simulink library "MBDS_Applications"  (R2018b)
settings: Solver=ode45  StartTime=0.0  StopTime=10.0  RelTol=1e-3
undefined symbols (not defined in the file or in its folder): Ts
libraries: KIBES_Signal x297, simulink x7
(part 5 of 6)

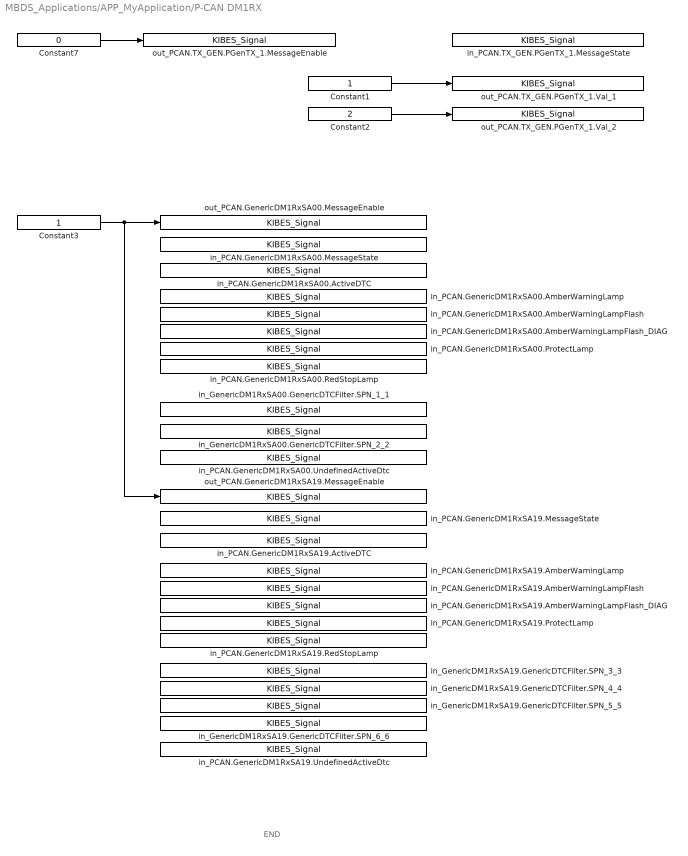
== system MBDS_Applications/APP_MyApplication/P-CAN DM1RX ==
  note: END
  Constant1 : Constant  InitFcn=|  OutDataTypeStr=uint8
      | if(exist('MBDS_BlockCallback', 'file'))
      |    MBDS_BlockCallback('Update', gcb);  
      | end
  Constant2 : Constant  InitFcn=|  Value=2  OutDataTypeStr=uint8
      | if(exist('MBDS_BlockCallback', 'file'))
      |    MBDS_BlockCallback('Update', gcb);  
      | end
  Constant3 : Constant  InitFcn=|  OutDataTypeStr=boolean
      | if(exist('MBDS_BlockCallback', 'file'))
      |    MBDS_BlockCallback('Update', gcb);  
      | end
  Constant7 : Constant  InitFcn=|  Value=0  OutDataTypeStr=boolean
      | if(exist('MBDS_BlockCallback', 'file'))
      |    MBDS_BlockCallback('Update', gcb);  
      | end
  in_GenericDM1RxSA00.GenericDTCFilter.SPN_1_1 : KIBES_Signal/KIBES_Signal  MBDS_LibraryBlock=on  DatabaseKey=293  SignalName=GenericDM1RxSA00.GenericDTCFilter.SPN_1_1  SymbolName=GenericDM1RxSA00_GenericDTCFilter_SPN_1_1_000293  DataType=boolean  Init=0  Slope=1  Bias=0  DataSize=1  fpDataType=boolean  BlockIOType=Inport  DeviceType=0
  in_GenericDM1RxSA00.GenericDTCFilter.SPN_2_2 : KIBES_Signal/KIBES_Signal  MBDS_LibraryBlock=on  DatabaseKey=294  SignalName=GenericDM1RxSA00.GenericDTCFilter.SPN_2_2  SymbolName=GenericDM1RxSA00_GenericDTCFilter_SPN_2_2_000294  DataType=boolean  Init=0  Slope=1  Bias=0  DataSize=1  fpDataType=boolean  BlockIOType=Inport  DeviceType=0
  in_GenericDM1RxSA19.GenericDTCFilter.SPN_3_3 : KIBES_Signal/KIBES_Signal  MBDS_LibraryBlock=on  DatabaseKey=290  SignalName=GenericDM1RxSA19.GenericDTCFilter.SPN_3_3  SymbolName=GenericDM1RxSA19_GenericDTCFilter_SPN_3_3_000290  DataType=boolean  Init=0  Slope=1  Bias=0  DataSize=1  fpDataType=boolean  BlockIOType=Inport  DeviceType=0
  in_GenericDM1RxSA19.GenericDTCFilter.SPN_4_4 : KIBES_Signal/KIBES_Signal  MBDS_LibraryBlock=on  DatabaseKey=291  SignalName=GenericDM1RxSA19.GenericDTCFilter.SPN_4_4  SymbolName=GenericDM1RxSA19_GenericDTCFilter_SPN_4_4_000291  DataType=boolean  Init=0  Slope=1  Bias=0  DataSize=1  fpDataType=boolean  BlockIOType=Inport  DeviceType=0
  in_GenericDM1RxSA19.GenericDTCFilter.SPN_5_5 : KIBES_Signal/KIBES_Signal  MBDS_LibraryBlock=on  DatabaseKey=296  SignalName=GenericDM1RxSA19.GenericDTCFilter.SPN_5_5  SymbolName=GenericDM1RxSA19_GenericDTCFilter_SPN_5_5_000296  DataType=boolean  Init=0  Slope=1  Bias=0  DataSize=1  fpDataType=boolean  BlockIOType=Inport  DeviceType=0
  in_GenericDM1RxSA19.GenericDTCFilter.SPN_6_6 : KIBES_Signal/KIBES_Signal  MBDS_LibraryBlock=on  DatabaseKey=303  SignalName=GenericDM1RxSA19.GenericDTCFilter.SPN_6_6  SymbolName=GenericDM1RxSA19_GenericDTCFilter_SPN_6_6_000303  DataType=boolean  Init=0  Slope=1  Bias=0  DataSize=1  fpDataType=boolean  BlockIOType=Inport  DeviceType=0
  in_PCAN.GenericDM1RxSA00.ActiveDTC : KIBES_Signal/KIBES_Signal  MBDS_LibraryBlock=on  DatabaseKey=274  SignalName=PCAN.GenericDM1RxSA00.ActiveDTC  SymbolName=PCAN_GenericDM1RxSA00_ActiveDTC_000274  DataType=boolean  Init=0  Slope=1  Bias=0  DataSize=1  fpDataType=boolean  BlockIOType=Inport  DeviceType=0
  in_PCAN.GenericDM1RxSA00.AmberWarningLamp : KIBES_Signal/KIBES_Signal  MBDS_LibraryBlock=on  DatabaseKey=275  SignalName=PCAN.GenericDM1RxSA00.AmberWarningLamp  SymbolName=PCAN_GenericDM1RxSA00_AmberWarningLamp_000275  DataType=boolean  Init=0  Slope=1  Bias=0  DataSize=1  fpDataType=boolean  BlockIOType=Inport  DeviceType=0
  in_PCAN.GenericDM1RxSA00.AmberWarningLampFlash : KIBES_Signal/KIBES_Signal  MBDS_LibraryBlock=on  DatabaseKey=276  SignalName=PCAN.GenericDM1RxSA00.AmberWarningLampFlash  SymbolName=PCAN_GenericDM1RxSA00_AmberWarningLampFlash_000276  DataType=uint8  Init=0  Slope=1  Bias=0  DataSize=1  fpDataType=uint8  BlockIOType=Inport  DeviceType=0
  in_PCAN.GenericDM1RxSA00.AmberWarningLampFlash_DIAG : KIBES_Signal/KIBES_Signal  MBDS_LibraryBlock=on  DatabaseKey=277  SignalName=PCAN.GenericDM1RxSA00.AmberWarningLampFlash_DIAG  SymbolName=PCAN_GenericDM1RxSA00_AmberWarningLampFlash_DIAG_000277  DataType=uint16  Init=1  Slope=1  Bias=0  DataSize=1  fpDataType=uint16  BlockIOType=Inport  DeviceType=0
  in_PCAN.GenericDM1RxSA00.MessageState : KIBES_Signal/KIBES_Signal  MBDS_LibraryBlock=on  DatabaseKey=279  SignalName=PCAN.GenericDM1RxSA00.MessageState  SymbolName=PCAN_GenericDM1RxSA00_MessageState_000279  DataType=uint16  Init=0  Slope=1  Bias=0  DataSize=1  fpDataType=uint16  BlockIOType=Inport  DeviceType=0
  in_PCAN.GenericDM1RxSA00.ProtectLamp : KIBES_Signal/KIBES_Signal  MBDS_LibraryBlock=on  DatabaseKey=280  SignalName=PCAN.GenericDM1RxSA00.ProtectLamp  SymbolName=PCAN_GenericDM1RxSA00_ProtectLamp_000280  DataType=boolean  Init=0  Slope=1  Bias=0  DataSize=1  fpDataType=boolean  BlockIOType=Inport  DeviceType=0
  in_PCAN.GenericDM1RxSA00.RedStopLamp : KIBES_Signal/KIBES_Signal  MBDS_LibraryBlock=on  DatabaseKey=281  SignalName=PCAN.GenericDM1RxSA00.RedStopLamp  SymbolName=PCAN_GenericDM1RxSA00_RedStopLamp_000281  DataType=boolean  Init=0  Slope=1  Bias=0  DataSize=1  fpDataType=boolean  BlockIOType=Inport  DeviceType=0
  in_PCAN.GenericDM1RxSA00.UndefinedActiveDtc : KIBES_Signal/KIBES_Signal  MBDS_LibraryBlock=on  DatabaseKey=403  SignalName=PCAN.GenericDM1RxSA00.UndefinedActiveDtc  SymbolName=PCAN_GenericDM1RxSA00_UndefinedActiveDtc_000403  DataType=boolean  Init=0  Slope=1  Bias=0  DataSize=1  fpDataType=boolean  BlockIOType=Inport  DeviceType=0
  in_PCAN.GenericDM1RxSA19.ActiveDTC : KIBES_Signal/KIBES_Signal  MBDS_LibraryBlock=on  DatabaseKey=282  SignalName=PCAN.GenericDM1RxSA19.ActiveDTC  SymbolName=PCAN_GenericDM1RxSA19_ActiveDTC_000282  DataType=boolean  Init=0  Slope=1  Bias=0  DataSize=1  fpDataType=boolean  BlockIOType=Inport  DeviceType=0
  in_PCAN.GenericDM1RxSA19.AmberWarningLamp : KIBES_Signal/KIBES_Signal  MBDS_LibraryBlock=on  DatabaseKey=283  SignalName=PCAN.GenericDM1RxSA19.AmberWarningLamp  SymbolName=PCAN_GenericDM1RxSA19_AmberWarningLamp_000283  DataType=boolean  Init=0  Slope=1  Bias=0  DataSize=1  fpDataType=boolean  BlockIOType=Inport  DeviceType=0
  in_PCAN.GenericDM1RxSA19.AmberWarningLampFlash : KIBES_Signal/KIBES_Signal  MBDS_LibraryBlock=on  DatabaseKey=284  SignalName=PCAN.GenericDM1RxSA19.AmberWarningLampFlash  SymbolName=PCAN_GenericDM1RxSA19_AmberWarningLampFlash_000284  DataType=uint8  Init=0  Slope=1  Bias=0  DataSize=1  fpDataType=uint8  BlockIOType=Inport  DeviceType=0
  in_PCAN.GenericDM1RxSA19.AmberWarningLampFlash_DIAG : KIBES_Signal/KIBES_Signal  MBDS_LibraryBlock=on  DatabaseKey=285  SignalName=PCAN.GenericDM1RxSA19.AmberWarningLampFlash_DIAG  SymbolName=PCAN_GenericDM1RxSA19_AmberWarningLampFlash_DIAG_000285  DataType=uint16  Init=1  Slope=1  Bias=0  DataSize=1  fpDataType=uint16  BlockIOType=Inport  DeviceType=0
  in_PCAN.GenericDM1RxSA19.MessageState : KIBES_Signal/KIBES_Signal  MBDS_LibraryBlock=on  DatabaseKey=287  SignalName=PCAN.GenericDM1RxSA19.MessageState  SymbolName=PCAN_GenericDM1RxSA19_MessageState_000287  DataType=uint16  Init=0  Slope=1  Bias=0  DataSize=1  fpDataType=uint16  BlockIOType=Inport  DeviceType=0
  in_PCAN.GenericDM1RxSA19.ProtectLamp : KIBES_Signal/KIBES_Signal  MBDS_LibraryBlock=on  DatabaseKey=288  SignalName=PCAN.GenericDM1RxSA19.ProtectLamp  SymbolName=PCAN_GenericDM1RxSA19_ProtectLamp_000288  DataType=boolean  Init=0  Slope=1  Bias=0  DataSize=1  fpDataType=boolean  BlockIOType=Inport  DeviceType=0
  in_PCAN.GenericDM1RxSA19.RedStopLamp : KIBES_Signal/KIBES_Signal  MBDS_LibraryBlock=on  DatabaseKey=289  SignalName=PCAN.GenericDM1RxSA19.RedStopLamp  SymbolName=PCAN_GenericDM1RxSA19_RedStopLamp_000289  DataType=boolean  Init=0  Slope=1  Bias=0  DataSize=1  fpDataType=boolean  BlockIOType=Inport  DeviceType=0
  in_PCAN.GenericDM1RxSA19.UndefinedActiveDtc : KIBES_Signal/KIBES_Signal  MBDS_LibraryBlock=on  DatabaseKey=404  SignalName=PCAN.GenericDM1RxSA19.UndefinedActiveDtc  SymbolName=PCAN_GenericDM1RxSA19_UndefinedActiveDtc_000404  DataType=boolean  Init=0  Slope=1  Bias=0  DataSize=1  fpDataType=boolean  BlockIOType=Inport  DeviceType=0
  in_PCAN.TX_GEN.PGenTX_1.MessageState : KIBES_Signal/KIBES_Signal  MBDS_LibraryBlock=on  DatabaseKey=260  SignalName=PCAN.TX_GEN.PGenTX_1.MessageState  SymbolName=PCAN_TX_GEN_PGenTX_1_MessageState_000260  DataType=uint16  Init=0  Slope=1  Bias=0  DataSize=1  fpDataType=uint16  BlockIOType=Inport  DeviceType=0
  out_PCAN.GenericDM1RxSA00.MessageEnable : KIBES_Signal/KIBES_Signal  MBDS_LibraryBlock=on  DatabaseKey=278  SignalName=PCAN.GenericDM1RxSA00.MessageEnable  SymbolName=PCAN_GenericDM1RxSA00_MessageEnable_000278  DataType=boolean  Init=0  Slope=1  Bias=0  DataSize=1  fpDataType=boolean  BlockIOType=Outport  DeviceType=0
  out_PCAN.GenericDM1RxSA19.MessageEnable : KIBES_Signal/KIBES_Signal  MBDS_LibraryBlock=on  DatabaseKey=286  SignalName=PCAN.GenericDM1RxSA19.MessageEnable  SymbolName=PCAN_GenericDM1RxSA19_MessageEnable_000286  DataType=boolean  Init=0  Slope=1  Bias=0  DataSize=1  fpDataType=boolean  BlockIOType=Outport  DeviceType=0
  out_PCAN.TX_GEN.PGenTX_1.MessageEnable : KIBES_Signal/KIBES_Signal  MBDS_LibraryBlock=on  DatabaseKey=259  SignalName=PCAN.TX_GEN.PGenTX_1.MessageEnable  SymbolName=PCAN_TX_GEN_PGenTX_1_MessageEnable_000259  DataType=boolean  Init=0  Slope=1  Bias=0  DataSize=1  fpDataType=boolean  BlockIOType=Outport  DeviceType=0
  out_PCAN.TX_GEN.PGenTX_1.Val_1 : KIBES_Signal/KIBES_Signal  MBDS_LibraryBlock=on  DatabaseKey=261  SignalName=PCAN.TX_GEN.PGenTX_1.Val_1  SymbolName=PCAN_TX_GEN_PGenTX_1_Val_1_000261  DataType=uint8  Init=0  Slope=1  Bias=0  DataSize=1  fpDataType=uint8  BlockIOType=Outport  DeviceType=0
  out_PCAN.TX_GEN.PGenTX_1.Val_2 : KIBES_Signal/KIBES_Signal  MBDS_LibraryBlock=on  DatabaseKey=262  SignalName=PCAN.TX_GEN.PGenTX_1.Val_2  SymbolName=PCAN_TX_GEN_PGenTX_1_Val_2_000262  DataType=uint8  Init=0  Slope=1  Bias=0  DataSize=1  fpDataType=uint8  BlockIOType=Outport  DeviceType=0
  wires:
  Constant3/1 -> out_PCAN.GenericDM1RxSA00.MessageEnable/1, out_PCAN.GenericDM1RxSA19.MessageEnable/1
  Constant2/1 -> out_PCAN.TX_GEN.PGenTX_1.Val_2/1
  Constant1/1 -> out_PCAN.TX_GEN.PGenTX_1.Val_1/1
  Constant7/1 -> out_PCAN.TX_GEN.PGenTX_1.MessageEnable/1

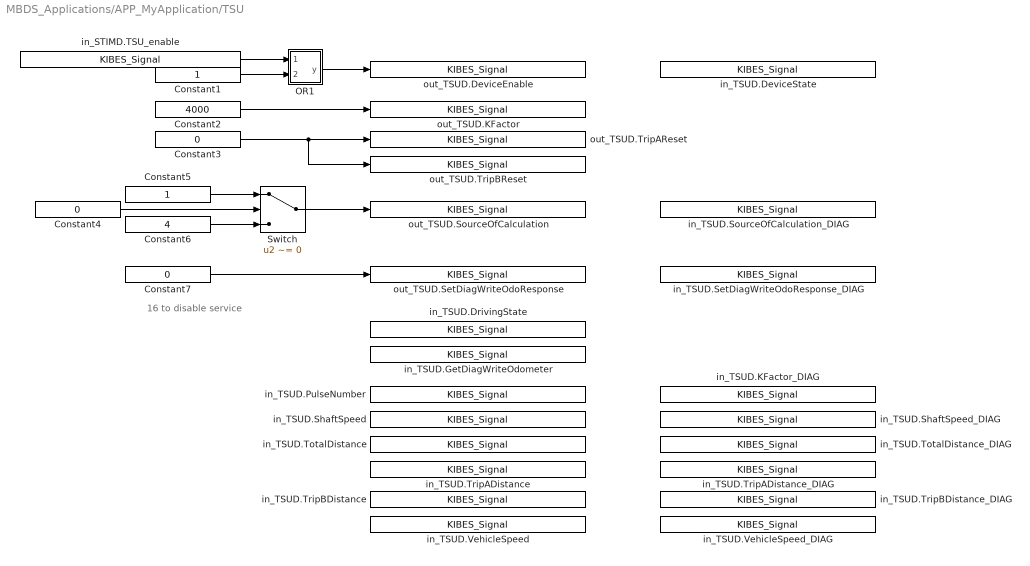
== system MBDS_Applications/APP_MyApplication/TSU ==
  note: 16 to disable service
  Constant1 : Constant  InitFcn=|  OutDataTypeStr=boolean
      | if(exist('MBDS_BlockCallback', 'file'))
      |    MBDS_BlockCallback('Update', gcb);  
      | end
  Constant2 : Constant  InitFcn=|  Value=4000  OutDataTypeStr=uint32
      | if(exist('MBDS_BlockCallback', 'file'))
      |    MBDS_BlockCallback('Update', gcb);  
      | end
  Constant3 : Constant  InitFcn=|  Value=0  OutDataTypeStr=boolean
      | if(exist('MBDS_BlockCallback', 'file'))
      |    MBDS_BlockCallback('Update', gcb);  
      | end
  Constant4 : Constant  InitFcn=|  Value=0  OutDataTypeStr=boolean
      | if(exist('MBDS_BlockCallback', 'file'))
      |    MBDS_BlockCallback('Update', gcb);  
      | end
  Constant5 : Constant  InitFcn=|  OutDataTypeStr=uint8
      | if(exist('MBDS_BlockCallback', 'file'))
      |    MBDS_BlockCallback('Update', gcb);  
      | end
  Constant6 : Constant  InitFcn=|  Value=4  OutDataTypeStr=uint8
      | if(exist('MBDS_BlockCallback', 'file'))
      |    MBDS_BlockCallback('Update', gcb);  
      | end
  Constant7 : Constant  InitFcn=|  Value=0  OutDataTypeStr=uint8
      | if(exist('MBDS_BlockCallback', 'file'))
      |    MBDS_BlockCallback('Update', gcb);  
      | end
  OR1 : Subsystem  InitFcn=|  mask(OR){MBDS_LibraryBlock=on, BitwiseMode=off, Inputs=2, UseBitMask=off, BitMask='A1', OutDataTypeStr=Inherit: Inherit via back propagation, MBDS_BlockVersion=07.21.05}
      | if(exist('MBDS_BlockCallback', 'file'))
      |    MBDS_BlockCallback('Update', gcb);
      | end
      mask prompts: MBDS_LibraryBlock "MBDS library block"; BitwiseMode "Use 'bitwise' mode"; Inputs "Number of input ports:"; UseBitMask "Use bit mask"; BitMask "Bit mask:"; OutDataTypeStr "Output data type:"; MBDS_BlockVersion "Version:"
      mask help: Logical or bitwise OR operator. For multiple inputs, operators are applied across the inputs. For a single input, operators are applied across the input vector. In bitwise mode a bit mask can be applied onto single input signals.
      mask init: same as MBDS_Applications/APP_MyApplication/NOT
      mask Help: eval(['open([workdir(''library_dir:''),''\Blockset\help\'',get_param(gcb,''MaskType''),''.html''])'])
      mask Callback BitwiseMode:
      | if(exist('MBDS_BlockCallback', 'file'))
      |    MBDS_BlockCallback('BitwiseMode', gcb);
      | end
      mask Callback Inputs:
      | if(exist('MBDS_BlockCallback', 'file'))
      |    MBDS_BlockCallback('Inputs', gcb);
      | end
      mask Callback UseBitMask:
      | if(exist('MBDS_BlockCallback', 'file'))
      |    MBDS_BlockCallback('UseBitMask', gcb);
      | end
      mask Callback BitMask:
      | if(exist('MBDS_BlockCallback', 'file'))
      |    MBDS_BlockCallback('BitMask', gcb);
      | end
      mask TypeOptions OutDataTypeStr: Inherit: Inherit via back propagation | int8 | uint8 | int16 | uint16 | int32 | uint32 | boolean
      mask Callback OutDataTypeStr:
      | % Adopt Value
      | if(exist('MBDS_BlockCallback', 'file'))
      |    MBDS_BlockCallback('OutDataTypeStr', gcb);
      | end
      mask DialogControl ParameterTabVar0 Prompt: Main
      mask DialogControl ParameterTabVar01 Prompt: Signal Attributes
      mask DialogControl ParameterTabVar012 Prompt: Version
      mask Display:
      | % Show icon or block text
      | if(UseBitMask)
      |    if(isnumeric(BitMask))
      |       BitMaskString = ['0x',dec2hex(floor(BitMask))];
      |    elseif(ischar(BitMask))
      |       BitMaskString = ['0x',upper(BitMask)];
      |    else
      |       BitMaskString = '???';
      |    end
      |    disp(sprintf(['OR\n', BitMaskString]))
      | else
      |    disp('OR')
      | end
  Switch : Switch  InitFcn=|  Criteria=u2 ~= 0  OutDataTypeStr=Inherit: Inherit via back propagation  mask(Switch){MBDS_LibraryBlock=on, OutDataTypeStr_=Inherit: Inherit via back propagation, SaturateOnIntegerOverflow_=off, InputSameDT_=off, MBDS_BlockVersion=07.21.05}
      | if(exist('MBDS_BlockCallback', 'file'))
      |    MBDS_BlockCallback('Update', gcb);  
      | end
      mask prompts: MBDS_LibraryBlock "MBDS library block"; OutDataTypeStr_ "Output data type:"; SaturateOnIntegerOverflow_ "Saturate on integer overflow"; InputSameDT_ "Require all inputs to have the same data type"; MBDS_BlockVersion "Block version:"
      mask help: Pass through input 1 when input 2 is not equal to zero; otherwise pass through input 3. The inputs are numbered top to bottom (or left to right). The first and third input ports are data ports, and the second input port is the control port.
      mask init: same as MBDS_Applications/APP_MyApplication/NOT
      mask Help: eval(['open([workdir(''library_dir:''),''\Blockset\help\'',get_param(gcb,''MaskType''),''.html''])'])
      mask TypeOptions OutDataTypeStr_: Inherit: Inherit via back propagation | single | int8 | uint8 | int16 | uint16 | int32 | uint32
      mask DialogControl ParameterTabVar0 Prompt: Signal Attributes
      mask DialogControl ParameterTabVar01 Prompt: Version
  in_STIMD.TSU_enable : KIBES_Signal/KIBES_Signal  MBDS_LibraryBlock=on  DatabaseKey=391  SignalName=STIMD.TSU_enable  SymbolName=STIMD_TSU_enable_000391  DataType=boolean  Init=0  Slope=1  Bias=0  DataSize=1  fpDataType=boolean  BlockIOType=Inport  DeviceType=2
  in_TSUD.DeviceState : KIBES_Signal/KIBES_Signal  MBDS_LibraryBlock=on  DatabaseKey=379  SignalName=TSUD.DeviceState  SymbolName=TSUD_DeviceState_000379  DataType=uint16  Init=0  Slope=1  Bias=0  DataSize=1  fpDataType=uint16  BlockIOType=Inport  DeviceType=0
  in_TSUD.DrivingState : KIBES_Signal/KIBES_Signal  MBDS_LibraryBlock=on  DatabaseKey=376  SignalName=TSUD.DrivingState  SymbolName=TSUD_DrivingState_000376  DataType=boolean  Init=0  Slope=1  Bias=0  DataSize=1  fpDataType=boolean  BlockIOType=Inport  DeviceType=0
  in_TSUD.GetDiagWriteOdometer : KIBES_Signal/KIBES_Signal  MBDS_LibraryBlock=on  DatabaseKey=383  SignalName=TSUD.GetDiagWriteOdometer  SymbolName=TSUD_GetDiagWriteOdometer_000383  DataType=boolean  Init=0  Slope=1  Bias=0  DataSize=1  fpDataType=boolean  BlockIOType=Inport  DeviceType=0
  in_TSUD.KFactor_DIAG : KIBES_Signal/KIBES_Signal  MBDS_LibraryBlock=on  DatabaseKey=375  SignalName=TSUD.KFactor_DIAG  SymbolName=TSUD_KFactor_DIAG_000375  DataType=uint16  Init=1  Slope=1  Bias=0  DataSize=1  fpDataType=uint16  BlockIOType=Inport  DeviceType=0
  in_TSUD.PulseNumber : KIBES_Signal/KIBES_Signal  MBDS_LibraryBlock=on  DatabaseKey=381  SignalName=TSUD.PulseNumber  SymbolName=TSUD_PulseNumber_000381  DataType=uint16  Init=0  Slope=1  Bias=0  DataSize=1  fpDataType=uint16  BlockIOType=Inport  DeviceType=0
  in_TSUD.SetDiagWriteOdoResponse_DIAG : KIBES_Signal/KIBES_Signal  MBDS_LibraryBlock=on  DatabaseKey=374  SignalName=TSUD.SetDiagWriteOdoResponse_DIAG  SymbolName=TSUD_SetDiagWriteOdoResponse_DIAG_000374  DataType=uint16  Init=1  Slope=1  Bias=0  DataSize=1  fpDataType=uint16  BlockIOType=Inport  DeviceType=0
  in_TSUD.ShaftSpeed : KIBES_Signal/KIBES_Signal  MBDS_LibraryBlock=on  DatabaseKey=382  SignalName=TSUD.ShaftSpeed  SymbolName=TSUD_ShaftSpeed_000382  DataType=uint16  Init=0  Slope=1  Bias=0  DataSize=1  fpDataType=uint16  BlockIOType=Inport  DeviceType=0
  in_TSUD.ShaftSpeed_DIAG : KIBES_Signal/KIBES_Signal  MBDS_LibraryBlock=on  DatabaseKey=370  SignalName=TSUD.ShaftSpeed_DIAG  SymbolName=TSUD_ShaftSpeed_DIAG_000370  DataType=uint16  Init=1  Slope=1  Bias=0  DataSize=1  fpDataType=uint16  BlockIOType=Inport  DeviceType=0
  in_TSUD.SourceOfCalculation_DIAG : KIBES_Signal/KIBES_Signal  MBDS_LibraryBlock=on  DatabaseKey=369  SignalName=TSUD.SourceOfCalculation_DIAG  SymbolName=TSUD_SourceOfCalculation_DIAG_000369  DataType=uint16  Init=1  Slope=1  Bias=0  DataSize=1  fpDataType=uint16  BlockIOType=Inport  DeviceType=0
  in_TSUD.TotalDistance : KIBES_Signal/KIBES_Signal  MBDS_LibraryBlock=on  DatabaseKey=384  SignalName=TSUD.TotalDistance  SymbolName=TSUD_TotalDistance_000384  DataType=uint32  Init=0  Slope=1  Bias=0  DataSize=1  fpDataType=uint32  BlockIOType=Inport  DeviceType=0
  in_TSUD.TotalDistance_DIAG : KIBES_Signal/KIBES_Signal  MBDS_LibraryBlock=on  DatabaseKey=368  SignalName=TSUD.TotalDistance_DIAG  SymbolName=TSUD_TotalDistance_DIAG_000368  DataType=uint16  Init=1  Slope=1  Bias=0  DataSize=1  fpDataType=uint16  BlockIOType=Inport  DeviceType=0
  in_TSUD.TripADistance : KIBES_Signal/KIBES_Signal  MBDS_LibraryBlock=on  DatabaseKey=378  SignalName=TSUD.TripADistance  SymbolName=TSUD_TripADistance_000378  DataType=uint32  Init=0  Slope=1  Bias=0  DataSize=1  fpDataType=uint32  BlockIOType=Inport  DeviceType=0
  in_TSUD.TripADistance_DIAG : KIBES_Signal/KIBES_Signal  MBDS_LibraryBlock=on  DatabaseKey=372  SignalName=TSUD.TripADistance_DIAG  SymbolName=TSUD_TripADistance_DIAG_000372  DataType=uint16  Init=1  Slope=1  Bias=0  DataSize=1  fpDataType=uint16  BlockIOType=Inport  DeviceType=0
  in_TSUD.TripBDistance : KIBES_Signal/KIBES_Signal  MBDS_LibraryBlock=on  DatabaseKey=377  SignalName=TSUD.TripBDistance  SymbolName=TSUD_TripBDistance_000377  DataType=uint32  Init=0  Slope=1  Bias=0  DataSize=1  fpDataType=uint32  BlockIOType=Inport  DeviceType=0
  in_TSUD.TripBDistance_DIAG : KIBES_Signal/KIBES_Signal  MBDS_LibraryBlock=on  DatabaseKey=373  SignalName=TSUD.TripBDistance_DIAG  SymbolName=TSUD_TripBDistance_DIAG_000373  DataType=uint16  Init=1  Slope=1  Bias=0  DataSize=1  fpDataType=uint16  BlockIOType=Inport  DeviceType=0
  in_TSUD.VehicleSpeed : KIBES_Signal/KIBES_Signal  MBDS_LibraryBlock=on  DatabaseKey=380  SignalName=TSUD.VehicleSpeed  SymbolName=TSUD_VehicleSpeed_000380  DataType=uint16  Init=0  Slope=1  Bias=0  DataSize=1  fpDataType=uint16  BlockIOType=Inport  DeviceType=0
  in_TSUD.VehicleSpeed_DIAG : KIBES_Signal/KIBES_Signal  MBDS_LibraryBlock=on  DatabaseKey=371  SignalName=TSUD.VehicleSpeed_DIAG  SymbolName=TSUD_VehicleSpeed_DIAG_000371  DataType=uint16  Init=1  Slope=1  Bias=0  DataSize=1  fpDataType=uint16  BlockIOType=Inport  DeviceType=0
  out_TSUD.DeviceEnable : KIBES_Signal/KIBES_Signal  MBDS_LibraryBlock=on  DatabaseKey=385  SignalName=TSUD.DeviceEnable  SymbolName=TSUD_DeviceEnable_000385  DataType=boolean  Init=0  Slope=1  Bias=0  DataSize=1  fpDataType=boolean  BlockIOType=Outport  DeviceType=0
  out_TSUD.KFactor : KIBES_Signal/KIBES_Signal  MBDS_LibraryBlock=on  DatabaseKey=387  SignalName=TSUD.KFactor  SymbolName=TSUD_KFactor_000387  DataType=uint32  Init=0  Slope=1  Bias=0  DataSize=1  fpDataType=uint32  BlockIOType=Outport  DeviceType=0
  out_TSUD.SetDiagWriteOdoResponse : KIBES_Signal/KIBES_Signal  MBDS_LibraryBlock=on  DatabaseKey=386  SignalName=TSUD.SetDiagWriteOdoResponse  SymbolName=TSUD_SetDiagWriteOdoResponse_000386  DataType=uint8  Init=0  Slope=1  Bias=0  DataSize=1  fpDataType=uint8  BlockIOType=Outport  DeviceType=0
  out_TSUD.SourceOfCalculation : KIBES_Signal/KIBES_Signal  MBDS_LibraryBlock=on  DatabaseKey=390  SignalName=TSUD.SourceOfCalculation  SymbolName=TSUD_SourceOfCalculation_000390  DataType=uint8  Init=0  Slope=1  Bias=0  DataSize=1  fpDataType=uint8  BlockIOType=Outport  DeviceType=0
  out_TSUD.TripAReset : KIBES_Signal/KIBES_Signal  MBDS_LibraryBlock=on  DatabaseKey=388  SignalName=TSUD.TripAReset  SymbolName=TSUD_TripAReset_000388  DataType=boolean  Init=0  Slope=1  Bias=0  DataSize=1  fpDataType=boolean  BlockIOType=Outport  DeviceType=0
  out_TSUD.TripBReset : KIBES_Signal/KIBES_Signal  MBDS_LibraryBlock=on  DatabaseKey=389  SignalName=TSUD.TripBReset  SymbolName=TSUD_TripBReset_000389  DataType=boolean  Init=0  Slope=1  Bias=0  DataSize=1  fpDataType=boolean  BlockIOType=Outport  DeviceType=0
  wires:
  Constant7/1 -> out_TSUD.SetDiagWriteOdoResponse/1
  Constant4/1 -> Switch/2
  Constant6/1 -> Switch/3
  Constant5/1 -> Switch/1
  Switch/1 -> out_TSUD.SourceOfCalculation/1
  Constant3/1 -> out_TSUD.TripAReset/1, out_TSUD.TripBReset/1
  Constant2/1 -> out_TSUD.KFactor/1
  OR1/1(y) -> out_TSUD.DeviceEnable/1
  in_STIMD.TSU_enable/1 -> OR1/1(u1)
  Constant1/1 -> OR1/2(u2)

== system MBDS_Applications/APP_MyApplication/TimerPulse ==
  note: Timer Pulse
  bo_Enable : Inport  OutDataTypeStr=boolean
  EdgeRising : Subsystem  InitFcn=|  mask(EdgeRising){MBDS_LibraryBlock=on, R_Enabled=off, IV_Enabled=off, IV=0, MBDS_BlockVersion=05.32}
      | if(exist('MBDS_BlockCallback', 'file'))
      |    MBDS_BlockCallback('Update', gcb);
      | end
      mask prompts: MBDS_LibraryBlock "MBDS library block"; R_Enabled "Show R port"; IV_Enabled "Show IV port"; IV "Initial value (IV):"; MBDS_BlockVersion "Block version:"
      mask help: The output indicates true if the input value changes from false to true.
      mask init: same as MBDS_Applications/APP_MyApplication/NOT
      mask Help: eval(['open([workdir(''library_dir:''),''\Blockset\help\'',get_param(gcb,''MaskType''),''.html''])'])
      mask Callback R_Enabled:
      | % Update mask parameter dialog
      | if(exist('MBDS_BlockCallback', 'file'))
      |    MBDS_BlockCallback('R_Enabled', gcb);
      | end
      mask Callback IV_Enabled:
      | % Update mask parameter dialog
      | if(exist('MBDS_BlockCallback', 'file'))
      |    MBDS_BlockCallback('IV_Enabled', gcb);
      | end
      mask Callback IV:
      | % Adopt Value
      | if(exist('MBDS_BlockCallback', 'file'))
      |    MBDS_BlockCallback('IV', gcb);
      | end
      mask DialogControl ParameterTabVar0 Prompt: Main
      mask DialogControl ParameterTabVar01 Prompt: Version
      mask Display:
      | % Show icon or block text
      | if(exist('EdgeRising.tif', 'file'))
      |    image('EdgeRising.tif', [0.295739348370927 0.17 0.378947368421053 0.66]);
      |    disp('')
      | else
      |    disp(sprintf('Rising\nEdge\nDetection'));
      | end
      | 
      | % Display port labels
      | port_label('input', 1, 'u');
      | port_label('output', 1, 'y');
  TimeSource : Subsystem  InitFcn=|  mask(TimeSource){MBDS_LibraryBlock=on, InputValue=5s, MBDS_BlockVersion=07.21.04}
      | if(exist('MBDS_BlockCallback', 'file'))
      |    MBDS_BlockCallback('Update', gcb);
      | end
      mask prompts: MBDS_LibraryBlock "MBDS Library Block"; InputValue "Constant value:"; MBDS_BlockVersion "Block version:"
      mask help: This block outputs a constant time signal based on a uint32 data type. Specify the time by the 'Constant value' parameter. Comply to the format: 1d2h3m4s5ms, for example 12d10h34m4s231ms, 1s500ms or 2h1s.
      mask init:
      | MBDS_BlockCallback('Copy', gcb);
      | Text = InputValue;
      | try
      |    % Try to evaluate project constant 
      |    EvalValue = evalin('base', InputValue);
      |    if(~isempty(EvalValue))
      |       InputValue = EvalValue;
      |    end
      | end
      | % Convert string to value (enable silent mode)
      | Value = ConvertSignalValue(InputValue, 'time', 'Str2Val', true);
      mask Help: eval(['open([workdir(''Library_Dir:''),''\Blockset\Help\'',get_param(gcb,''MaskType''),''.html''])'])
      mask DialogControl ParameterTabVar0 Prompt: Main
      mask DialogControl ParameterTabVar01 Prompt: Version
      mask Display: disp([' ',Text,' ']);
  Timer_RE1 : Subsystem  InitFcn=|  mask(Timer_RE){MBDS_LibraryBlock=on, dT_Enabled=off, dT=1000*Ts, E_Enabled=off, R_Enabled=on, IV_Enabled=on, IV=0, y_Enabled=on, x_Enabled=off, OutDataTypeStr=Inherit: Inherit via back propagation, MBDS_BlockVersion=05.20}
      | if(exist('MBDS_BlockCallback', 'file'))
      |    MBDS_BlockCallback('Update', gcb);
      | end
      mask prompts: MBDS_LibraryBlock "MBDS library block"; dT_Enabled "Show dT port"; dT "Sample rate (dT):"; E_Enabled "Show E port"; R_Enabled "Show R port"; IV_Enabled "Show IV port"; IV "Initial value (IV):"; y_Enabled "Show y port"; x_Enabled "Show x port"; OutDataTypeStr "Output data type:"; MBDS_BlockVersion "Block version:"
      mask help: The block indicates true, if the initial time IV has not passed since the last reset of the block. Reset can only be performed, if the counter has run down to zero.
      mask init: same as MBDS_Applications/APP_MyApplication/NOT
      settings: AttributesFormatString=dT = %<dT>
      mask Help: eval(['open([workdir(''library_dir:''),''\Blockset\help\'',get_param(gcb,''MaskType''),''.html''])'])
      mask Callback dT_Enabled:
      | % Update mask parameter dialog
      | if(exist('MBDS_BlockCallback', 'file'))
      |    MBDS_BlockCallback('dT_Enabled', gcb);
      | end
      mask Callback dT:
      | % Adopt Value
      | if(exist('MBDS_BlockCallback', 'file'))
      |    MBDS_BlockCallback('dT', gcb);
      | end
      mask Callback R_Enabled:
      | % Update mask parameter dialog
      | if(exist('MBDS_BlockCallback', 'file'))
      |    MBDS_BlockCallback('R_Enabled', gcb);
      | end
      mask Callback IV_Enabled:
      | % Update mask parameter dialog
      | if(exist('MBDS_BlockCallback', 'file'))
      |    MBDS_BlockCallback('IV_Enabled', gcb);
      | end
      mask Callback IV:
      | % Adopt Value
      | if(exist('MBDS_BlockCallback', 'file'))
      |    MBDS_BlockCallback('IV', gcb);
      | end
      mask Callback y_Enabled:
      | % Update mask parameter dialog
      | if(exist('MBDS_BlockCallback', 'file'))
      |    MBDS_BlockCallback('y_Enabled', gcb);
      | end
      mask Callback x_Enabled:
      | % Update mask parameter dialog
      | if(exist('MBDS_BlockCallback', 'file'))
      |    MBDS_BlockCallback('x_Enabled', gcb);
      | end
      mask TypeOptions OutDataTypeStr: Inherit: Inherit via back propagation | int8 | uint8 | int16 | uint16 | int32 | uint32
      mask Callback OutDataTypeStr:
      | % Configure data type
      | if(exist('MBDS_BlockCallback', 'file'))
      |    MBDS_BlockCallback('OutDataTypeStr', gcb);
      | end
      mask DialogControl ParameterTabVar0 Prompt: Main
      mask DialogControl ParameterTabVar01 Prompt: Signal Attributes
      mask DialogControl ParameterTabVar012 Prompt: Version
      mask Display:
      | % Show icon or block text
      | if(exist('Timer.tif', 'file'))
      |    image('Timer.tif', [0.295739348370927 0.17 0.378947368421053 0.66]);
      |    disp('')
      | else
      |    disp(sprintf('Timer'));
      | end
      | 
      | % Display port labels
      | port_label('input', 1, 'R');
      | port_label('input', 2, 'IV');
      | port_label('output', 1, 'y');
  bo_Pulse : Outport
  wires:
  TimeSource/1(Out) -> Timer_RE1/2(IV)
  bo_Enable/1 -> EdgeRising/1(u)
  Timer_RE1/1(y) -> bo_Pulse/1
  EdgeRising/1(y) -> Timer_RE1/1(R)

== system MBDS_Applications/APP_MyApplication/DM13/OR1 ==
  note: OR
  u1 : Inport  OutDataTypeStr=boolean
  u2 : Inport  Port=2  OutDataTypeStr=boolean
  DataType : DataTypeConversion  OutDataTypeStr=boolean
  Operator : Logic  Operator=OR  AllPortsSameDT=off  OutDataTypeStr=boolean
  y : Outport
  wires:
  DataType/1 -> y/1
  u2/1 -> Operator/2
  u1/1 -> Operator/1
  Operator/1 -> DataType/1

== system MBDS_Applications/APP_MyApplication/DM2_3_11/OR1 ==
  note: OR
  u1 : Inport  OutDataTypeStr=boolean
  u2 : Inport  Port=2  OutDataTypeStr=boolean
  DataType : DataTypeConversion  OutDataTypeStr=boolean
  Operator : Logic  Operator=OR  AllPortsSameDT=off  OutDataTypeStr=boolean
  y : Outport
  wires:
  DataType/1 -> y/1
  u2/1 -> Operator/2
  u1/1 -> Operator/1
  Operator/1 -> DataType/1

== system MBDS_Applications/APP_MyApplication/DM2_3_11/OR2 ==
  note: OR
  u1 : Inport  OutDataTypeStr=boolean
  u2 : Inport  Port=2  OutDataTypeStr=boolean
  DataType : DataTypeConversion  OutDataTypeStr=boolean
  Operator : Logic  Operator=OR  AllPortsSameDT=off  OutDataTypeStr=boolean
  y : Outport
  wires:
  DataType/1 -> y/1
  u2/1 -> Operator/2
  u1/1 -> Operator/1
  Operator/1 -> DataType/1

== system MBDS_Applications/APP_MyApplication/DM2_3_11/OR3 ==
  note: OR
  u1 : Inport  OutDataTypeStr=boolean
  u2 : Inport  Port=2  OutDataTypeStr=boolean
  DataType : DataTypeConversion  OutDataTypeStr=boolean
  Operator : Logic  Operator=OR  AllPortsSameDT=off  OutDataTypeStr=boolean
  y : Outport
  wires:
  DataType/1 -> y/1
  u2/1 -> Operator/2
  u1/1 -> Operator/1
  Operator/1 -> DataType/1

== system MBDS_Applications/APP_MyApplication/DTC/GetBit ==
  note: GetBit
  u : Inport
  SEL : Inport  Port=2
  LoopOverBits : Subsystem
  y : Outport
  wires:
  LoopOverBits/1(y) -> y/1
  SEL/1 -> LoopOverBits/2(SEL)
  u/1 -> LoopOverBits/1(u)

== system MBDS_Applications/APP_MyApplication/DTC/GetBit1 ==
  note: GetBit
  u : Inport
  SEL : Inport  Port=2
  LoopOverBits : Subsystem
  y : Outport
  wires:
  LoopOverBits/1(y) -> y/1
  SEL/1 -> LoopOverBits/2(SEL)
  u/1 -> LoopOverBits/1(u)

== system MBDS_Applications/APP_MyApplication/DTC/GetBit2 ==
  note: GetBit
  u : Inport
  SEL : Inport  Port=2
  LoopOverBits : Subsystem
  y : Outport
  wires:
  LoopOverBits/1(y) -> y/1
  SEL/1 -> LoopOverBits/2(SEL)
  u/1 -> LoopOverBits/1(u)

== system MBDS_Applications/APP_MyApplication/DTC/GetBit3 ==
  note: GetBit
  u : Inport
  SEL : Inport  Port=2
  LoopOverBits : Subsystem
  y : Outport
  wires:
  LoopOverBits/1(y) -> y/1
  SEL/1 -> LoopOverBits/2(SEL)
  u/1 -> LoopOverBits/1(u)

== system MBDS_Applications/APP_MyApplication/DTC/GetBit4 ==
  note: GetBit
  u : Inport
  SEL : Inport  Port=2
  LoopOverBits : Subsystem
  y : Outport
  wires:
  LoopOverBits/1(y) -> y/1
  SEL/1 -> LoopOverBits/2(SEL)
  u/1 -> LoopOverBits/1(u)

== system MBDS_Applications/APP_MyApplication/DTC/GetBit5 ==
  note: GetBit
  u : Inport
  SEL : Inport  Port=2
  LoopOverBits : Subsystem
  y : Outport
  wires:
  LoopOverBits/1(y) -> y/1
  SEL/1 -> LoopOverBits/2(SEL)
  u/1 -> LoopOverBits/1(u)

== system MBDS_Applications/APP_MyApplication/DTC/GetBit6 ==
  note: GetBit
  u : Inport
  SEL : Inport  Port=2
  LoopOverBits : Subsystem
  y : Outport
  wires:
  LoopOverBits/1(y) -> y/1
  SEL/1 -> LoopOverBits/2(SEL)
  u/1 -> LoopOverBits/1(u)

== system MBDS_Applications/APP_MyApplication/DTC/OR ==
  note: OR
  u1 : Inport  OutDataTypeStr=boolean
  u2 : Inport  Port=2  OutDataTypeStr=boolean
  DataType : DataTypeConversion  OutDataTypeStr=boolean
  Operator : Logic  Operator=OR  AllPortsSameDT=off  OutDataTypeStr=boolean
  y : Outport
  wires:
  DataType/1 -> y/1
  u2/1 -> Operator/2
  u1/1 -> Operator/1
  Operator/1 -> DataType/1

== system MBDS_Applications/APP_MyApplication/DTC/OR1 ==
  note: OR
  u1 : Inport  OutDataTypeStr=boolean
  u2 : Inport  Port=2  OutDataTypeStr=boolean
  DataType : DataTypeConversion  OutDataTypeStr=boolean
  Operator : Logic  Operator=OR  AllPortsSameDT=off  OutDataTypeStr=boolean
  y : Outport
  wires:
  DataType/1 -> y/1
  u2/1 -> Operator/2
  u1/1 -> Operator/1
  Operator/1 -> DataType/1

== system MBDS_Applications/APP_MyApplication/DTC/OR2 ==
  note: OR
  u1 : Inport  OutDataTypeStr=boolean
  u2 : Inport  Port=2  OutDataTypeStr=boolean
  DataType : DataTypeConversion  OutDataTypeStr=boolean
  Operator : Logic  Operator=OR  AllPortsSameDT=off  OutDataTypeStr=boolean
  y : Outport
  wires:
  DataType/1 -> y/1
  u2/1 -> Operator/2
  u1/1 -> Operator/1
  Operator/1 -> DataType/1

== system MBDS_Applications/APP_MyApplication/DTC List/OR1 ==
  note: OR
  u1 : Inport  OutDataTypeStr=boolean
  u2 : Inport  Port=2  OutDataTypeStr=boolean
  DataType : DataTypeConversion  OutDataTypeStr=boolean
  Operator : Logic  Operator=OR  AllPortsSameDT=off  OutDataTypeStr=boolean
  y : Outport
  wires:
  DataType/1 -> y/1
  u2/1 -> Operator/2
  u1/1 -> Operator/1
  Operator/1 -> DataType/1

== system MBDS_Applications/APP_MyApplication/DateTime/DateTimeAssemble ==
  note: DateTimeAssemble
  Year : Inport  OutDataTypeStr=uint16
  Month : Inport  Port=2  OutDataTypeStr=uint8
  Day : Inport  Port=3  OutDataTypeStr=uint8
  Hours : Inport  Port=4  OutDataTypeStr=uint8
  Minutes : Inport  Port=5  OutDataTypeStr=uint8
  Seconds : Inport  Port=6  OutDataTypeStr=uint8
  CheckIfInputIsValid : Subsystem
  ConvertToDateTime : Subsystem
  ConvertToNrOfDays : Subsystem
  DT : Outport  OutDataTypeStr=uint32
  ENO : Outport  Port=2  OutDataTypeStr=boolean
  wires:
  CheckIfInputIsValid/7(bo_ENO) -> ENO/1
  CheckIfInputIsValid/1(u8_Seconds) -> ConvertToDateTime/1(u8_Seconds)
  CheckIfInputIsValid/2(u8_Minutes) -> ConvertToDateTime/2(u8_Minutes)
  CheckIfInputIsValid/3(u8_Hours) -> ConvertToDateTime/3(u8_Hours)
  CheckIfInputIsValid/4(u8_Day) -> ConvertToNrOfDays/1(u8_Day)
  CheckIfInputIsValid/5(u8_Month) -> ConvertToNrOfDays/2(u8_Month)
  CheckIfInputIsValid/6(u16_Year) -> ConvertToNrOfDays/3(u16_Year)
  Year/1 -> CheckIfInputIsValid/6(u16_YearIn)
  Month/1 -> CheckIfInputIsValid/5(u8_MonthIn)
  Day/1 -> CheckIfInputIsValid/4(u8_DayIn)
  Hours/1 -> CheckIfInputIsValid/3(u8_HoursIn)
  Minutes/1 -> CheckIfInputIsValid/2(u8_MinutesIn)
  Seconds/1 -> CheckIfInputIsValid/1(u8_SecondsIn)
  ConvertToDateTime/1(u32_DateTime) -> DT/1
  ConvertToNrOfDays/1(u16_NrOfDays) -> ConvertToDateTime/4(u16_NrOfDays)

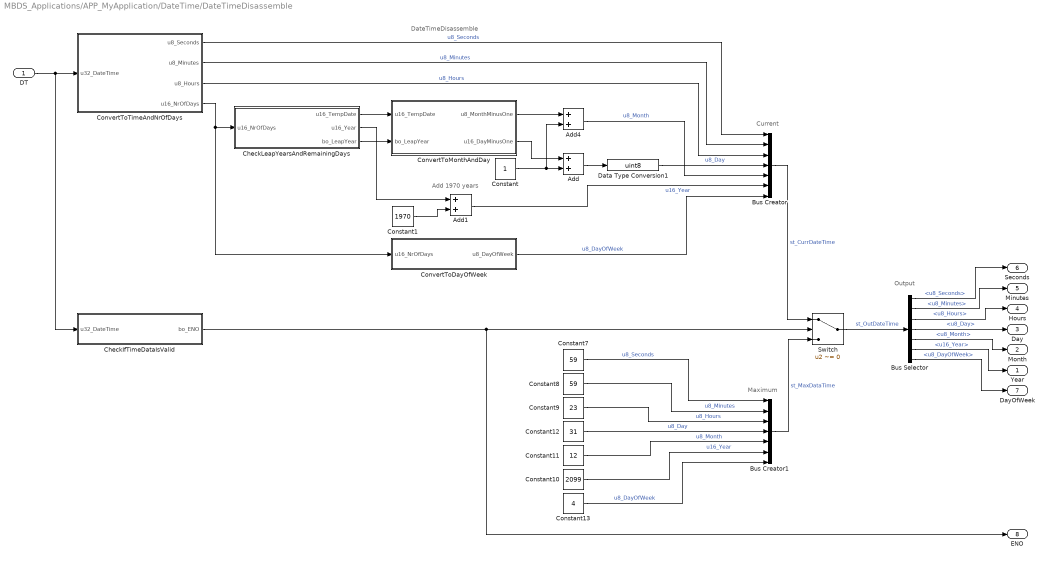
== system MBDS_Applications/APP_MyApplication/DateTime/DateTimeDisassemble ==
  note: DateTimeDisassemble
  note: Add 1970 years
  note: Current
  note: Maximum
  note: Output
  DT : Inport  OutDataTypeStr=uint32
  Add : Sum  OutDataTypeStr=uint32
  Add1 : Sum  OutDataTypeStr=uint16
  Add4 : Sum  OutDataTypeStr=uint8
  Bus Creator : BusCreator  Inputs='u8_Seconds','u8_Minutes','u8_Hours','u8_Day','u8_Month','u16_Year','u8_DayOfWeek'
  Bus Creator1 : BusCreator  Inputs=7
  Bus Selector : BusSelector  OutputSignals=u8_Seconds,u8_Minutes,u8_Hours,u8_Day,u8_Month,u16_Year,u8_DayOfWeek
  CheckIfTimeDataIsValid : Subsystem
  CheckLeapYearsAndRemainingDays : Subsystem
  Constant : Constant  OutDataTypeStr=uint8
  Constant1 : Constant  Value=1970  OutDataTypeStr=uint16
  Constant10 : Constant  Value=2099  OutDataTypeStr=uint16
  Constant11 : Constant  Value=12  OutDataTypeStr=uint8
  Constant12 : Constant  Value=31  OutDataTypeStr=uint8
  Constant13 : Constant  Value=4  OutDataTypeStr=uint8
  Constant7 : Constant  Value=59  OutDataTypeStr=uint8
  Constant8 : Constant  Value=59  OutDataTypeStr=uint8
  Constant9 : Constant  Value=23  OutDataTypeStr=uint8
  ConvertToDayOfWeek : Subsystem
  ConvertToMonthAndDay : Subsystem  TreatAsAtomicUnit=on
  ConvertToTimeAndNrOfDays : Subsystem
  Data Type Conversion1 : DataTypeConversion  OutDataTypeStr=uint8
  Switch : Switch  Criteria=u2 ~= 0
  Year : Outport  OutDataTypeStr=uint16
  Month : Outport  Port=2  OutDataTypeStr=uint8
  Day : Outport  Port=3  OutDataTypeStr=uint8
  Hours : Outport  Port=4  OutDataTypeStr=uint8
  Minutes : Outport  Port=5  OutDataTypeStr=uint8
  Seconds : Outport  Port=6  OutDataTypeStr=uint8
  DayOfWeek : Outport  Port=7  OutDataTypeStr=uint8
  ENO : Outport  Port=8  OutDataTypeStr=boolean
  wires:
  CheckIfTimeDataIsValid/1(bo_ENO) -> Switch/2, ENO/1
  CheckLeapYearsAndRemainingDays/1(u16_TempDate) -> ConvertToMonthAndDay/1(u16_TempDate)
  ConvertToDayOfWeek/1(u8_DayOfWeek) -> Bus Creator/7  "u8_DayOfWeek"
  Constant/1 -> Add/2, Add4/2
  ConvertToTimeAndNrOfDays/4(u16_NrOfDays) -> CheckLeapYearsAndRemainingDays/1(u16_NrOfDays), ConvertToDayOfWeek/1(u16_NrOfDays)
  Bus Selector/7 -> DayOfWeek/1  "<u8_DayOfWeek>"
  Constant10/1 -> Bus Creator1/6  "u16_Year"
  Constant12/1 -> Bus Creator1/4  "u8_Day"
  Bus Selector/6 -> Year/1  "<u16_Year>"
  Data Type Conversion1/1 -> Bus Creator/4  "u8_Day"
  Bus Selector/4 -> Day/1  "<u8_Day>"
  Constant13/1 -> Bus Creator1/7  "u8_DayOfWeek"
  Constant11/1 -> Bus Creator1/5  "u8_Month"
  Constant9/1 -> Bus Creator1/3  "u8_Hours"
  Constant8/1 -> Bus Creator1/2  "u8_Minutes"
  Constant7/1 -> Bus Creator1/1  "u8_Seconds"
  Bus Creator1/1 -> Switch/3  "st_MaxDataTime"
  Switch/1 -> Bus Selector/1  "st_OutDateTime"
  Bus Creator/1 -> Switch/1  "st_CurrDateTime"
  Bus Selector/5 -> Month/1  "<u8_Month>"
  Bus Selector/3 -> Hours/1  "<u8_Hours>"
  Bus Selector/2 -> Minutes/1  "<u8_Minutes>"
  Bus Selector/1 -> Seconds/1  "<u8_Seconds>"
  Add4/1 -> Bus Creator/5  "u8_Month"
  ConvertToMonthAndDay/1(u8_MonthMinusOne) -> Add4/1
  Add/1 -> Data Type Conversion1/1
  DT/1 -> ConvertToTimeAndNrOfDays/1(u32_DateTime), CheckIfTimeDataIsValid/1(u32_DateTime)
  CheckLeapYearsAndRemainingDays/3(bo_LeapYear) -> ConvertToMonthAndDay/2(bo_LeapYear)
  Constant1/1 -> Add1/2
  CheckLeapYearsAndRemainingDays/2(u16_Year) -> Add1/1
  ConvertToMonthAndDay/2(u16_DayMinusOne) -> Add/1
  ConvertToTimeAndNrOfDays/2(u8_Minutes) -> Bus Creator/2  "u8_Minutes"
  ConvertToTimeAndNrOfDays/3(u8_Hours) -> Bus Creator/3  "u8_Hours"
  ConvertToTimeAndNrOfDays/1(u8_Seconds) -> Bus Creator/1  "u8_Seconds"
  Add1/1 -> Bus Creator/6  "u16_Year"

== system MBDS_Applications/APP_MyApplication/TSU/OR1 ==
  note: OR
  u1 : Inport  OutDataTypeStr=boolean
  u2 : Inport  Port=2  OutDataTypeStr=boolean
  DataType : DataTypeConversion  OutDataTypeStr=boolean
  Operator : Logic  Operator=OR  AllPortsSameDT=off  OutDataTypeStr=boolean
  y : Outport
  wires:
  DataType/1 -> y/1
  u2/1 -> Operator/2
  u1/1 -> Operator/1
  Operator/1 -> DataType/1

== system MBDS_Applications/APP_MyApplication/TimerPulse/EdgeRising ==
  note: EdgeRising
  u : Inport  OutDataTypeStr=boolean
  Data Type Duplicate : DataTypeDuplicate
  IV : Constant  Value=0  OutDataTypeStr=Inherit: Inherit via back propagation
  NoReset : Subsystem
  R : Constant  Value=0  OutDataTypeStr=boolean
  Relational Operator : RelationalOperator  Operator=<  OutDataTypeStr=boolean  RndMeth=Nearest  InputSameDT=on
  Unit Delay : UnitDelay  SampleTime=-1
  y : Outport
  wires:
  Relational Operator/1 -> y/1
  Unit Delay/1 -> NoReset/3(u)
  NoReset/1(y) -> Relational Operator/1
  R/1 -> NoReset/2(Unused2)
  u/1 -> Data Type Duplicate/1, Relational Operator/2, Unit Delay/1
  IV/1 -> Data Type Duplicate/2, NoReset/1(Unused1)

== system MBDS_Applications/APP_MyApplication/TimerPulse/TimeSource ==
  note: TimeSource
  Constant : Constant  Value=Value  OutDataTypeStr=uint32  LockScale=on
  Out : Outport
  wires:
  Constant/1 -> Out/1

== system MBDS_Applications/APP_MyApplication/TimerPulse/Timer_RE1 ==
  note: Timer_RE
  R : Inport  OutDataTypeStr=boolean
  IV : Inport  Port=2
  Constant : Constant  Value=0  OutDataTypeStr=Inherit: Inherit via back propagation
  Constant1 : Constant  Value=0  OutDataTypeStr=Inherit: Inherit via back propagation
  Constant2 : Constant  Value=0  OutDataTypeStr=Inherit: Inherit via back propagation
  Data Type Duplicate : DataTypeDuplicate  NumInputPorts=3
  DoubleReset : Subsystem
  E : Constant  OutDataTypeStr=boolean
  NoEnable : Subsystem
  Relational Operator : RelationalOperator  Operator=<=  OutDataTypeStr=boolean  RndMeth=Nearest
  Relational Operator1 : RelationalOperator  Operator=>  OutDataTypeStr=boolean  RndMeth=Nearest
  Relational Operator2 : RelationalOperator  Operator=>  OutDataTypeStr=boolean  RndMeth=Nearest  InputSameDT=on
  Subtract : Sum  Inputs=+-  OutDataTypeStr=Inherit: Inherit via back propagation
  Switch1 : Switch  Criteria=u2 ~= 0  OutDataTypeStr=Inherit: Inherit via back propagation
  Unit Delay : UnitDelay  SampleTime=-1
  dT : Constant  Value=1000*Ts  OutDataTypeStr=Inherit: Inherit via back propagation
  x : Terminator
  y : Outport
  wires:
  Relational Operator2/1 -> y/1
  NoEnable/1(y) -> DoubleReset/4(u)
  Constant1/1 -> Relational Operator/2
  Unit Delay/1 -> Data Type Duplicate/2, Relational Operator/1, Subtract/1, Relational Operator1/1, NoEnable/3(Unused2)
  dT/1 -> Relational Operator1/2, Subtract/2
  Switch1/1 -> NoEnable/1(u)
  Relational Operator1/1 -> Switch1/2
  Subtract/1 -> Switch1/1
  Constant/1 -> Switch1/3
  Constant2/1 -> Relational Operator2/2
  DoubleReset/1(y) -> Data Type Duplicate/3, x/1, Unit Delay/1, Relational Operator2/1
  Relational Operator/1 -> DoubleReset/3(R2)
  IV/1 -> DoubleReset/1(IV), Data Type Duplicate/1
  E/1 -> NoEnable/2(Unused1)
  R/1 -> DoubleReset/2(R1)

== system MBDS_Applications/APP_MyApplication/DTC/GetBit/LoopOverBits ==
  note: No saturation
      | needed !
  note: Determine bit value
  note: Generate bit mask
  u : Inport
  SEL : Inport  Port=2
  Assignment1 : Assignment  IndexMode=Zero-based  IndexOptions=Index vector (port)  Indices=1  OutputSizes=[1 1]
  Bitwise Operator1 : simulink/Logic and Bit Operations/Bitwise Operator  logicop=AND  UseBitMask=off  NumInputPorts=2  BitMask=bin2dec('11011001')  BitMaskRealWorld=Stored Integer
  Constant2 : Constant  Value=0  OutDataTypeStr=Inherit: Inherit via back propagation
  Constant3 : Constant  OutDataTypeStr=Inherit: Inherit via back propagation
  Data Type Duplicate : DataTypeDuplicate  InitFcn=|
      | try
      |    MBDS_BlockCallback('Update', gcb);
      | end
  DataType : DataTypeConversion  OutDataTypeStr=boolean
  DataType1 : DataTypeConversion  OutDataTypeStr=uint8
  For Iterator : ForIterator  IterationSource=external  IndexMode=Zero-based  IterationVariableDataType=int8
  IndexOffset : Constant  Value=0  OutDataTypeStr=Inherit: Inherit via back propagation
  Relational Operator : RelationalOperator  Operator=~=  OutDataTypeStr=boolean  RndMeth=Nearest
  Selector : Selector  IndexMode=Zero-based  IndexOptions=Index vector (port)  Indices=[1 3]  OutputSizes=1
  Shift Arithmetic : ArithShift  BitShiftNumberSource=Input port  BitShiftNumber=8  BitShiftDirection=Left
      settings: InputPortMap=u0,p1
  Subtract : Sum  Inputs=+-  OutDataTypeStr=Inherit: Inherit via back propagation  InputSameDT=on
  Width : Width  DataType=uint8
  y : Outport
  wires:
  u/1 -> Data Type Duplicate/1, Bitwise Operator1/1
  DataType1/1 -> Selector/1
  SEL/1 -> Width/1, DataType/1, DataType1/1
  DataType/1 -> Assignment1/1
  Assignment1/1 -> y/1
  Relational Operator/1 -> Assignment1/2
  Constant2/1 -> Relational Operator/2
  Bitwise Operator1/1 -> Relational Operator/1
  Shift Arithmetic/1 -> Bitwise Operator1/2
  Constant3/1 -> Data Type Duplicate/2, Shift Arithmetic/1
  Width/1 -> For Iterator/1
  For Iterator/1 -> Assignment1/3, Selector/2
  Selector/1 -> Subtract/1
  Subtract/1 -> Shift Arithmetic/2
  IndexOffset/1 -> Subtract/2

== system MBDS_Applications/APP_MyApplication/DTC/GetBit1/LoopOverBits ==
  note: No saturation
      | needed !
  note: Determine bit value
  note: Generate bit mask
  u : Inport
  SEL : Inport  Port=2
  Assignment1 : Assignment  IndexMode=Zero-based  IndexOptions=Index vector (port)  Indices=1  OutputSizes=[1 1]
  Bitwise Operator1 : simulink/Logic and Bit Operations/Bitwise Operator  logicop=AND  UseBitMask=off  NumInputPorts=2  BitMask=bin2dec('11011001')  BitMaskRealWorld=Stored Integer
  Constant2 : Constant  Value=0  OutDataTypeStr=Inherit: Inherit via back propagation
  Constant3 : Constant  OutDataTypeStr=Inherit: Inherit via back propagation
  Data Type Duplicate : DataTypeDuplicate  InitFcn=|
      | try
      |    MBDS_BlockCallback('Update', gcb);
      | end
  DataType : DataTypeConversion  OutDataTypeStr=boolean
  DataType1 : DataTypeConversion  OutDataTypeStr=uint8
  For Iterator : ForIterator  IterationSource=external  IndexMode=Zero-based  IterationVariableDataType=int8
  IndexOffset : Constant  Value=0  OutDataTypeStr=Inherit: Inherit via back propagation
  Relational Operator : RelationalOperator  Operator=~=  OutDataTypeStr=boolean  RndMeth=Nearest
  Selector : Selector  IndexMode=Zero-based  IndexOptions=Index vector (port)  Indices=[1 3]  OutputSizes=1
  Shift Arithmetic : ArithShift  BitShiftNumberSource=Input port  BitShiftNumber=8  BitShiftDirection=Left
      settings: InputPortMap=u0,p1
  Subtract : Sum  Inputs=+-  OutDataTypeStr=Inherit: Inherit via back propagation  InputSameDT=on
  Width : Width  DataType=uint8
  y : Outport
  wires:
  u/1 -> Data Type Duplicate/1, Bitwise Operator1/1
  DataType1/1 -> Selector/1
  SEL/1 -> Width/1, DataType/1, DataType1/1
  DataType/1 -> Assignment1/1
  Assignment1/1 -> y/1
  Relational Operator/1 -> Assignment1/2
  Constant2/1 -> Relational Operator/2
  Bitwise Operator1/1 -> Relational Operator/1
  Shift Arithmetic/1 -> Bitwise Operator1/2
  Constant3/1 -> Data Type Duplicate/2, Shift Arithmetic/1
  Width/1 -> For Iterator/1
  For Iterator/1 -> Assignment1/3, Selector/2
  Selector/1 -> Subtract/1
  Subtract/1 -> Shift Arithmetic/2
  IndexOffset/1 -> Subtract/2

== system MBDS_Applications/APP_MyApplication/DTC/GetBit2/LoopOverBits ==
  note: No saturation
      | needed !
  note: Determine bit value
  note: Generate bit mask
  u : Inport
  SEL : Inport  Port=2
  Assignment1 : Assignment  IndexMode=Zero-based  IndexOptions=Index vector (port)  Indices=1  OutputSizes=[1 1]
  Bitwise Operator1 : simulink/Logic and Bit Operations/Bitwise Operator  logicop=AND  UseBitMask=off  NumInputPorts=2  BitMask=bin2dec('11011001')  BitMaskRealWorld=Stored Integer
  Constant2 : Constant  Value=0  OutDataTypeStr=Inherit: Inherit via back propagation
  Constant3 : Constant  OutDataTypeStr=Inherit: Inherit via back propagation
  Data Type Duplicate : DataTypeDuplicate  InitFcn=|
      | try
      |    MBDS_BlockCallback('Update', gcb);
      | end
  DataType : DataTypeConversion  OutDataTypeStr=boolean
  DataType1 : DataTypeConversion  OutDataTypeStr=uint8
  For Iterator : ForIterator  IterationSource=external  IndexMode=Zero-based  IterationVariableDataType=int8
  IndexOffset : Constant  Value=0  OutDataTypeStr=Inherit: Inherit via back propagation
  Relational Operator : RelationalOperator  Operator=~=  OutDataTypeStr=boolean  RndMeth=Nearest
  Selector : Selector  IndexMode=Zero-based  IndexOptions=Index vector (port)  Indices=[1 3]  OutputSizes=1
  Shift Arithmetic : ArithShift  BitShiftNumberSource=Input port  BitShiftNumber=8  BitShiftDirection=Left
      settings: InputPortMap=u0,p1
  Subtract : Sum  Inputs=+-  OutDataTypeStr=Inherit: Inherit via back propagation  InputSameDT=on
  Width : Width  DataType=uint8
  y : Outport
  wires:
  u/1 -> Data Type Duplicate/1, Bitwise Operator1/1
  DataType1/1 -> Selector/1
  SEL/1 -> Width/1, DataType/1, DataType1/1
  DataType/1 -> Assignment1/1
  Assignment1/1 -> y/1
  Relational Operator/1 -> Assignment1/2
  Constant2/1 -> Relational Operator/2
  Bitwise Operator1/1 -> Relational Operator/1
  Shift Arithmetic/1 -> Bitwise Operator1/2
  Constant3/1 -> Data Type Duplicate/2, Shift Arithmetic/1
  Width/1 -> For Iterator/1
  For Iterator/1 -> Assignment1/3, Selector/2
  Selector/1 -> Subtract/1
  Subtract/1 -> Shift Arithmetic/2
  IndexOffset/1 -> Subtract/2
